simulink model "Control_While_exp2"  (R2015b)
settings: Solver=VariableStepAuto  StartTime=0.0  StopTime=10.0  RelTol=1e-3
StartFcn:
  | open_scope
libraries: simulink x1
settings Model: Creator=LUBO  LastModifiedBy=LUBO

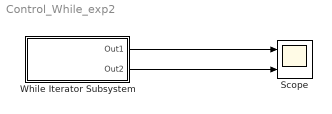
== system Control_While_exp2 ==
  Scope : Scope  NumInputPorts=2
  While Iterator Subsystem : Subsystem  TreatAsAtomicUnit=on
  wires:
  While Iterator Subsystem/1(Out1) -> Scope/1
  While Iterator Subsystem/2(Out2) -> Scope/2

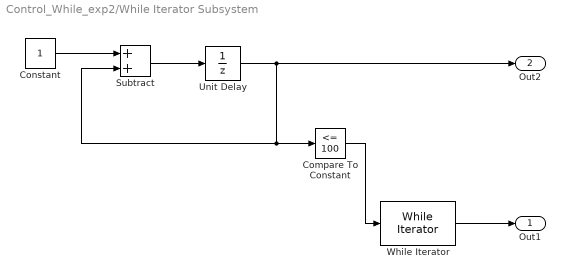
== system Control_While_exp2/While Iterator Subsystem ==
  Compare To Constant : simulink/Logic and Bit Operations/Compare To Constant  relop=<=  const=100  OutDataTypeStr=boolean
  Constant : Constant
  Subtract : Sum
  Unit Delay : UnitDelay  SampleTime=-1
  While Iterator : WhileIterator  WhileBlockType=do-while  ShowIterationPort=on
  Out1 : Outport
  Out2 : Outport  Port=2
  wires:
  While Iterator/1 -> Out1/1
  Constant/1 -> Subtract/1
  Subtract/1 -> Unit Delay/1
  Unit Delay/1 -> Subtract/2, Compare To Constant/1, Out2/1
  Compare To Constant/1 -> While Iterator/1
